simulink model "SRM_IOT"  (R2024b)
settings: Solver=VariableStepAuto  StartTime=0.0  StopTime=10.0  RelTol=1e-3
undefined symbols (not defined in the file): Ion, Lithium, sigbuilder_block
libraries: spsBreakerLib x120, spsSeriesRLCBranchLib x70, spsBatteryLib x42, spsIdealSwitchLib x33, spsVoltageMeasurementLib x27, slpidlib x17, spsMosfetLib x17, spsPWMGeneratorDCDCLib x11, spsDiodeLib x6, spsCurrentMeasurementLib x4, spsIGBTLib x2, spsThreePhaseSeriesRLCLoadLib x2
(part 1 of 5)
settings Model: SimulationMode=accelerator  Creator=Jatay  LastModifiedBy=Jatay

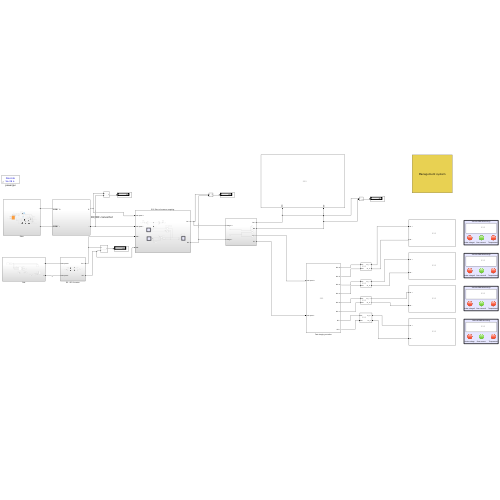
[thumbnail: Simulink's stored preview of the top-level diagram]
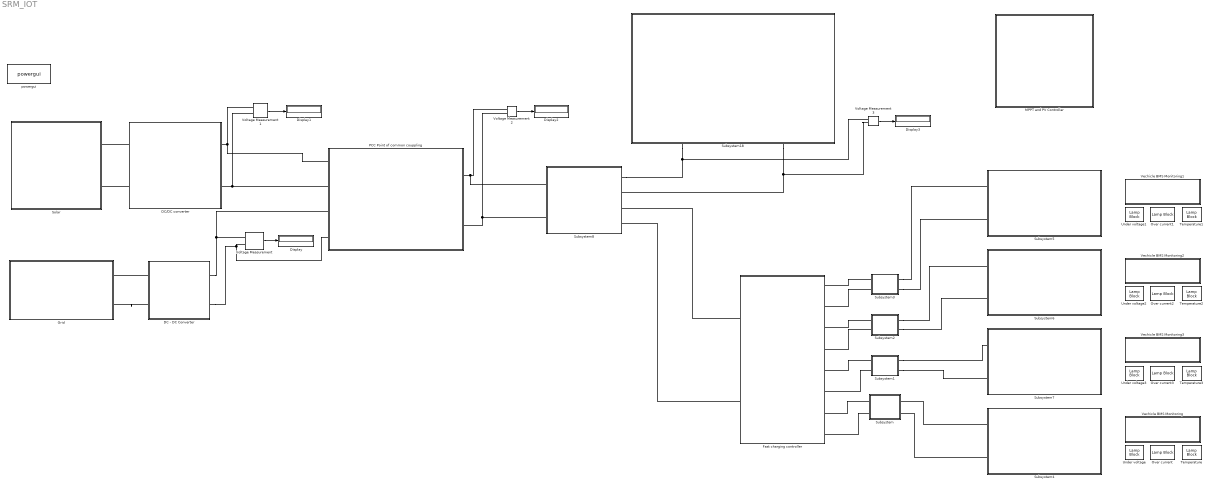
== system SRM_IOT ==
  DC - DC Converter : Subsystem
  DC/DC converter : Subsystem
  Display{,1..3} (4 alike) : Display
  Fast charging controller : Subsystem
      mask Display: image('FC.jpeg');
  Grid : Subsystem
  MPPT and PV Controller : Subsystem
      mask Display: disp('Management system')
  Over current{,1..3} (4 alike) : LampBlock  LabelPosition=Hide
  PCC Point of common couppling : Subsystem
  Solar : Subsystem
  Subsystem : Subsystem
      mask Display: image('plugin.jpeg');
  Subsystem1 : Subsystem
      mask Display: image('plugin.jpeg');
  Subsystem18 : Subsystem
      mask Display: image('swapping.webp');
  Subsystem2 : Subsystem
      mask Display: image('plugin.jpeg');
  Subsystem3 : Subsystem
      mask Display: image('plugin.jpeg');
  Subsystem4 : Subsystem
      mask Display: image('ev-1.jpeg');
  Subsystem5 : Subsystem
      mask Display: image('ev-1.jpeg');
  Subsystem6 : Subsystem
      mask Display: image('ev-1.jpeg');
  Subsystem7 : Subsystem
      mask Display: image('ev-1.jpeg');
  Subsystem8 : Subsystem
  Temperature{,1..3} (4 alike) : LampBlock  LabelPosition=Hide
  Under voltage{,1..3} (4 alike) : LampBlock  LabelPosition=Hide
  Vechicle BMS Monitoring : Subsystem
      mask Display: image('Dash_board.jpeg');
  Vechicle BMS Monitoring1 : Subsystem
      mask Display: image('Dash_board.jpeg');
  Vechicle BMS Monitoring2 : Subsystem
      mask Display: image('Dash_board.jpeg');
  Vechicle BMS Monitoring3 : Subsystem
      mask Display: image('Dash_board.jpeg');
  Voltage Measurement{,1..3} (4 alike) : spsVoltageMeasurementLib/Voltage Measurement  PhasorSimulation=off  OutputType=Complex  PSBequivalent=0
  powergui : sps_lib/powergui  Priority=1  SimulationMode=Discrete  SampleTime=5e-6  frequency=60  Iterations=50  frequencyindice=0  Pbase=100e6  ErrMax=1e-4  UnitsV=kV  UnitsW=MW  buscounter=0  FunctionMessages=off  echomessages=off  EnableUseOfTLC=off  CurrentSourceSwitches=off  DisableSnubberDevices=off  DisableRonSwitches=off  DisableVfSwitches=off  DisplayEquations=off  AutomaticDiscreteSolvers=off  SolverType=Tustin  Interpol=off  ExternalGateDelay=off  methode=off  Ts=0  x0status=blocks  SPID=off  SwTol=0  HookPort=off  NonlinearTolerance=1e-4  nMaxIteration=100  ContinueOnMaxIteration=off  RestoreLinks=warning  ResistiveCurrentMeasurement=off  Frange=[0:2:500]  Ylog=off  Xlog=on  ShowGrid=off  save=off  variable=ZData  structure=0  ZoomFFT=off  StartTime=0.0  cycles=1  DisplayStyle=1  fundamental=60  FreqAxis=off  MaxFrequency=1000  frequencyindicesteady=1  RmsSteady=1  display=off
  wires:
  Voltage Measurement/1 -> Display/1
  Voltage Measurement1/1 -> Display1/1
  Voltage Measurement2/1 -> Display2/1
  Voltage Measurement3/1 -> Display3/1
  connections:
  DC - DC Converter/LConn1 -- Grid/RConn1
  DC - DC Converter/RConn2 -- PCC Point of common couppling/LConn4 -- Voltage Measurement/LConn2
  DC - DC Converter/LConn2 -- Grid/RConn2
  DC - DC Converter/RConn1 -- PCC Point of common couppling/LConn3 -- Voltage Measurement/LConn1
  DC/DC converter/LConn2 -- Solar/RConn2
  DC/DC converter/LConn1 -- Solar/RConn1
  Voltage Measurement1/LConn1 -- PCC Point of common couppling/LConn1 -- DC/DC converter/RConn1
  Voltage Measurement1/LConn2 -- PCC Point of common couppling/LConn2 -- DC/DC converter/RConn2
  Voltage Measurement2/LConn1 -- Subsystem8/LConn1 -- PCC Point of common couppling/RConn1
  Voltage Measurement2/LConn2 -- PCC Point of common couppling/RConn2 -- Subsystem8/LConn2
  Subsystem18/LConn1 -- Subsystem8/RConn1 -- Voltage Measurement3/LConn1
  Subsystem18/LConn2 -- Subsystem8/RConn2 -- Voltage Measurement3/LConn2
  Subsystem3/RConn2 -- Subsystem5/LConn2
  Subsystem4/LConn1 -- Subsystem/RConn1
  Subsystem4/LConn2 -- Subsystem/RConn2
  Subsystem1/RConn1 -- Subsystem7/LConn1
  Subsystem2/RConn2 -- Subsystem6/LConn2
  Subsystem2/RConn1 -- Subsystem6/LConn1
  Subsystem3/RConn1 -- Subsystem5/LConn1
  Subsystem1/RConn2 -- Subsystem7/LConn2
  Fast charging controller/LConn2 -- Subsystem8/RConn3
  Fast charging controller/LConn1 -- Subsystem8/RConn4
  Subsystem3/LConn1 -- Fast charging controller/RConn8
  Subsystem3/LConn2 -- Fast charging controller/RConn7
  Subsystem2/LConn1 -- Fast charging controller/RConn6
  Subsystem2/LConn2 -- Fast charging controller/RConn5
  Subsystem1/LConn1 -- Fast charging controller/RConn4
  Subsystem1/LConn2 -- Fast charging controller/RConn3
  Subsystem/LConn1 -- Fast charging controller/RConn2
  Subsystem/LConn2 -- Fast charging controller/RConn1

== system SRM_IOT/DC - DC Converter ==
  C : spsSeriesRLCBranchLib/Series RLC Branch  LConnTagsString=__new0  RConnTagsString=__new0  BranchType=C  Resistance=0.01  Inductance=1e-3  SetiL0=off  InitialCurrent=0  Capacitance=1000e-6  Setx0=on  InitialVoltage=200  Measurements=None
  Diode : spsDiodeLib/Diode  Ron=0.001  Lon=0  Vf=1.1  IC=0  UseSnubber=off  Rs=500  Cs=250e-9  Measurements=off
  Diode2 : spsDiodeLib/Diode  Ron=0.001  Lon=0  Vf=0.7  IC=0  UseSnubber=off  Rs=500  Cs=250e-9  Measurements=off
  Display1 : Display
  Display2 : Display
  IGBT : spsIGBTLib/IGBT  Ron=0.001  Lon=0  Vf=1.1  Tf=1e-6  Tt=2e-6  IC=0  Rs=1e5  Cs=inf  Measurements=off
  Pulse Generator : DiscretePulseGenerator  PulseType=Time based  Period=10  PulseWidth=5
  RL : spsSeriesRLCBranchLib/Series RLC Branch  LConnTagsString=__new0  RConnTagsString=__new0  BranchType=RL  Resistance=0.05  Inductance=470e-6  SetiL0=off  InitialCurrent=0  Capacitance=1e-6  Setx0=off  InitialVoltage=0  Measurements=None
  Voltage Measurement1 : spsVoltageMeasurementLib/Voltage Measurement  PhasorSimulation=off  OutputType=Complex  PSBequivalent=0
  Voltage Measurement2 : spsVoltageMeasurementLib/Voltage Measurement  PhasorSimulation=off  OutputType=Complex  PSBequivalent=0
  DC + : PMIOPort  Side=Right
  solar panel + : PMIOPort  Port=2  Side=Left
  solar panel - : PMIOPort  Port=3  Side=Left
  DC - : PMIOPort  Port=4  Side=Right
  wires:
  Pulse Generator/1 -> IGBT/1
  Voltage Measurement1/1 -> Display1/1
  Voltage Measurement2/1 -> Display2/1
  connections:
  DC +/RConn1 -- Diode/RConn1 -- Voltage Measurement2/LConn1
  Diode2/RConn1 -- C/LConn1 -- RL/LConn1
  Diode/LConn1 -- RL/RConn1 -- IGBT/LConn1
  Diode2/LConn1 -- solar panel +/RConn1 -- Voltage Measurement1/LConn1
  DC -/RConn1 -- C/RConn1 -- Voltage Measurement1/LConn2 -- solar panel -/RConn1 -- IGBT/RConn1 -- Voltage Measurement2/LConn2

== system SRM_IOT/DC//DC converter ==
  DC - DC Converter : Subsystem
  DC bus : Subsystem
  Display : Display
  Voltage Measurement : spsVoltageMeasurementLib/Voltage Measurement  PhasorSimulation=off  OutputType=Complex  PSBequivalent=0
  Voltage Measurement2 : spsVoltageMeasurementLib/Voltage Measurement  PhasorSimulation=off  OutputType=Complex  PSBequivalent=0
  solar + : PMIOPort  Side=Left
  solar - : PMIOPort  Port=2  Side=Left
  + : PMIOPort  Port=3  Side=Right
  - : PMIOPort  Port=4  Side=Right
  tag scope: solar_controller=global
  wires:
  Voltage Measurement2/1 -> [solar_controller]
  Voltage Measurement/1 -> Display/1
  connections:
  DC - DC Converter/RConn1 -- DC bus/LConn1
  solar +/RConn1 -- DC - DC Converter/LConn1 -- Voltage Measurement2/LConn1
  DC - DC Converter/LConn2 -- Voltage Measurement2/LConn2 -- solar -/RConn1
  DC - DC Converter/RConn2 -- DC bus/LConn2
  -/RConn1 -- DC bus/RConn2 -- Voltage Measurement/LConn2
  Voltage Measurement/LConn1 -- DC bus/RConn1 -- +/RConn1

== system SRM_IOT/Fast charging controller ==
  note: Solar
  Fast charging Switching controller : Subsystem
  Ideal Switch{,1..3} (4 alike) : spsIdealSwitchLib/Ideal Switch  Ron=0.001  Lon=0  IC=0  Rs=1e5  Cs=inf  Measurements=off
  solar panel - : PMIOPort  Side=Left
  solar panel + : PMIOPort  Port=2  Side=Left
  DC + : PMIOPort  Port=3  Side=Right
  DC - : PMIOPort  Port=4  Side=Right
  DC +1 : PMIOPort  Port=5  Side=Right
  DC +2 : PMIOPort  Port=6  Side=Right
  DC +3 : PMIOPort  Port=7  Side=Right
  DC +4 : PMIOPort  Port=8  Side=Right
  DC +5 : PMIOPort  Port=9  Side=Right
  DC +6 : PMIOPort  Port=10  Side=Right
  wires:
  [gg1] -> Ideal Switch3/1
  [gg2] -> Ideal Switch2/1
  [gg3] -> Ideal Switch1/1
  [gg4] -> Ideal Switch/1
  connections:
  Ideal Switch3/LConn1 -- Ideal Switch2/LConn1 -- Ideal Switch1/LConn1 -- Ideal Switch/LConn1 -- solar panel +/RConn1
  solar panel -/RConn1 -- DC +5/RConn1 -- DC +4/RConn1 -- DC +2/RConn1 -- DC -/RConn1
  Ideal Switch3/RConn1 -- DC +/RConn1
  Ideal Switch2/RConn1 -- DC +1/RConn1
  Ideal Switch1/RConn1 -- DC +3/RConn1
  Ideal Switch/RConn1 -- DC +6/RConn1

== system SRM_IOT/Grid ==
  Display : Display
  Grid : spsThreePhaseSourceLib/Three-Phase Source  InternalConnection=Yg  VoltagePhases=off  Voltage=380  PhaseAngle=0  Voltage_phases=[25e3 25e3 25e3]/sqrt(3)  PhaseAngles_phases=[0 -120 +120]  Frequency=50  NonIdealSource=on  SpecifyImpedance=on  Resistance=0.8929  Inductance=16.58e-3  ShortCircuitLevel=100e6  BaseVoltage=380  XRratio=7  BusType=swing  Pref=10e3  Qref=0  Prefabc=[10e3, 10e3, 10e3]  Qrefabc=[0, 0, 0]  Qmin=-inf  Qmax=inf
  LOAD1 : spsThreePhaseSeriesRLCLoadLib/Three-Phase Series RLC Load  LConnTagsString=A|B|C  Configuration=Y (grounded)  NominalVoltage=380  Vabc=[1e3 1e3 1e3]  Vabcp=[1e3 1e3 1e3]  NominalFrequency=50  UnbalancedPower=off  ActivePower=1e3  InductivePower=0  CapacitivePower=0  Pabc=[10e3 9e3 11e3]  QLabc=[100 90 110]  QCabc=[100 90 110]  Pabcp=[10e3 9e3 11e3]  QLabcp=[100 90 110]  QCabcp=[100 90 110]  Measurements=None  LoadType=constant Z
  Measurement : spsThreePhaseVIMeasurementLib/Three-Phase V-I Measurement  VoltageMeasurement=phase-to-phase  SetLabelV=on  LabelV=Vabc_grid  Vpu=off  VpuLL=off  CurrentMeasurement=yes  SetLabelI=on  LabelI=Iabc_grid  Ipu=off  Pbase=100e6  Vbase=500e3  OutputType=Complex  PhasorSimulation=off  PSBequivalent=0
  Mux : Mux  Inputs=2
  Repeating Sequence Stair : simulink/Sources/Repeating Sequence Stair  OutValues=[0 0 1 1 0].'  tsamp=0.1  OutMin=[]  OutMax=[]  OutDataTypeStr=double  OutputDataTypeScalingMode=double  OutDataType=fixdt(0,8)  ConRadixGroup=Best Precision: Vector-wise  OutScaling=2^-12
  Scope : Scope
  Scope1 : Scope
  Scope2 : Scope  NumInputPorts=2
  V2G & G2V results : Scope  NumInputPorts=3
  Voltage Measurement : spsVoltageMeasurementLib/Voltage Measurement  PhasorSimulation=off  OutputType=Complex  PSBequivalent=0
  Wall charger Connection Box : Subsystem
  + : PMIOPort  Side=Right
  +1 : PMIOPort  Port=2  Side=Right
  tag scope: Control=global
  wires:
  [Control] -> Wall charger Connection Box/1(Control)
  Mux/1 -> V2G & G2V results/3
  [Vabc_grid] -> V2G & G2V results/1
  [Vabc_inv] -> V2G & G2V results/2
  Repeating Sequence Stair/1 -> [Control], Scope1/1
  [Vabc_inv] -> Mux/2
  [Iabc_out] -> Scope2/2
  [Iabc_inv] -> Scope/1
  [Vabc_out] -> Scope2/1
  Voltage Measurement/1 -> Display/1
  [Vabc_grid] -> Mux/1
  connections:
  Wall charger Connection Box/RConn2 -- Voltage Measurement/LConn2 -- +1/RConn1
  Grid/RConn1 -- Measurement/LConn1
  Grid/RConn3 -- Measurement/LConn3
  Wall charger Connection Box/RConn1 -- Voltage Measurement/LConn1 -- +/RConn1
  Grid/RConn2 -- Measurement/LConn2
  LOAD1/LConn3 -- Measurement/RConn3 -- Wall charger Connection Box/LConn3
  Measurement/RConn2 -- LOAD1/LConn2 -- Wall charger Connection Box/LConn2
  Measurement/RConn1 -- LOAD1/LConn1 -- Wall charger Connection Box/LConn1

== system SRM_IOT/MPPT and PV Controller ==
  Inverter controller : Subsystem
  Swapping battery controller : Subsystem

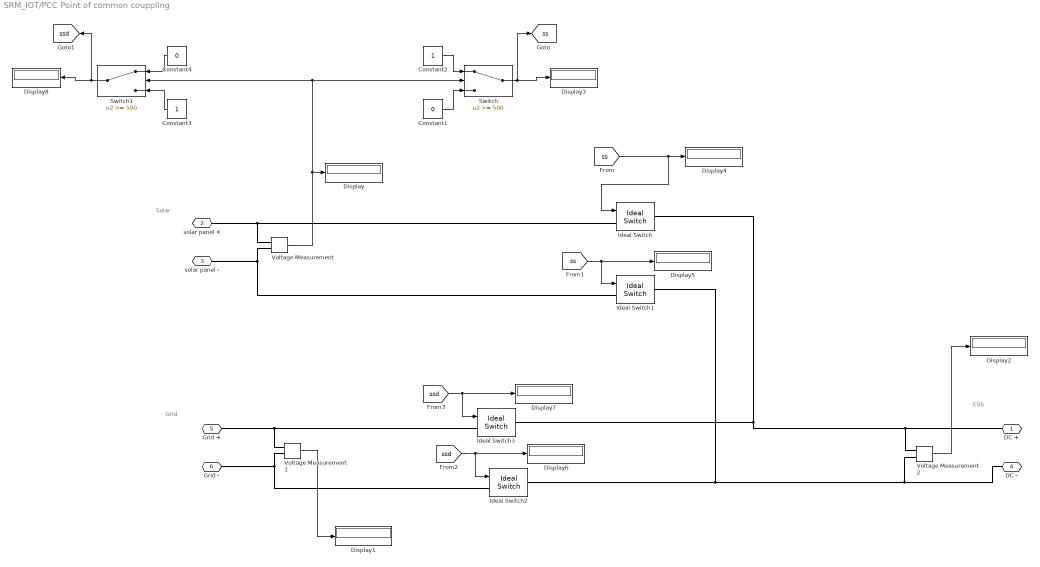
== system SRM_IOT/PCC Point of common couppling ==
  note: ESS
  note: Grid
  note: Solar
  Constant1 : Constant  Value=0
  Constant2 : Constant
  Constant3 : Constant
  Constant4 : Constant  Value=0
  Display{,1..8} (9 alike) : Display
  Ideal Switch{,1..3} (4 alike) : spsIdealSwitchLib/Ideal Switch  Ron=0.001  Lon=0  IC=0  Rs=1e5  Cs=inf  Measurements=off
  Switch : Switch  Threshold=500  SaturateOnIntegerOverflow=off  InputSameDT=off
  Switch1 : Switch  Threshold=500  SaturateOnIntegerOverflow=off  InputSameDT=off
  Voltage Measurement : spsVoltageMeasurementLib/Voltage Measurement  PhasorSimulation=off  OutputType=Complex  PSBequivalent=0
  Voltage Measurement1 : spsVoltageMeasurementLib/Voltage Measurement  PhasorSimulation=off  OutputType=Complex  PSBequivalent=0
  Voltage Measurement2 : spsVoltageMeasurementLib/Voltage Measurement  PhasorSimulation=off  OutputType=Complex  PSBequivalent=0
  DC + : PMIOPort  Side=Right
  solar panel + : PMIOPort  Port=2  Side=Left
  solar panel - : PMIOPort  Port=3  Side=Left
  DC - : PMIOPort  Port=4  Side=Right
  Grid + : PMIOPort  Port=5  Side=Left
  Grid - : PMIOPort  Port=6  Side=Left
  tag scope: ss=global, ssd=global
  wires:
  Voltage Measurement1/1 -> Display1/1
  Voltage Measurement2/1 -> Display2/1
  Switch/1 -> Display3/1, [ss]
  Constant2/1 -> Switch/1
  Constant1/1 -> Switch/3
  [ss] -> Ideal Switch/1, Display4/1
  [ss] -> Ideal Switch1/1, Display5/1
  [ssd] -> Ideal Switch2/1, Display6/1
  [ssd] -> Ideal Switch3/1, Display7/1
  Constant3/1 -> Switch1/3
  Voltage Measurement/1 -> Switch/2, Switch1/2, Display/1
  Constant4/1 -> Switch1/1
  Switch1/1 -> Display8/1, [ssd]
  connections:
  Voltage Measurement2/LConn2 -- Ideal Switch1/RConn1 -- Ideal Switch2/RConn1 -- DC -/RConn1
  Voltage Measurement2/LConn1 -- Ideal Switch3/RConn1 -- Ideal Switch/RConn1 -- DC +/RConn1
  Voltage Measurement/LConn1 -- solar panel +/RConn1 -- Ideal Switch/LConn1
  Voltage Measurement/LConn2 -- Ideal Switch1/LConn1 -- solar panel -/RConn1
  Voltage Measurement1/LConn2 -- Ideal Switch2/LConn1 -- Grid -/RConn1
  Grid +/RConn1 -- Ideal Switch3/LConn1 -- Voltage Measurement1/LConn1

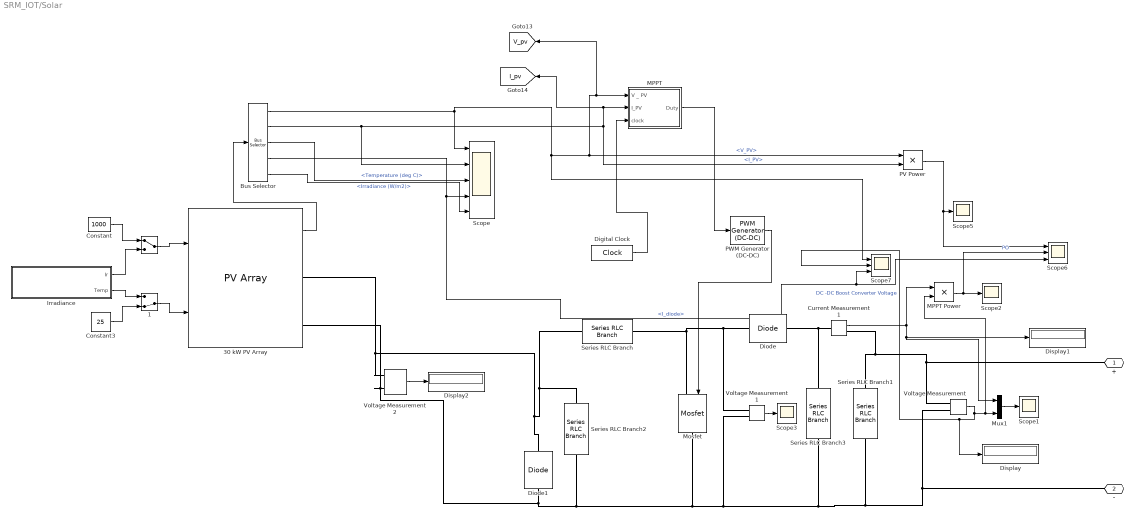
== system SRM_IOT/Solar ==
  "      " : ManualSwitch
  "      1" : ManualSwitch  CurrentSetting=0
  30 kW PV Array : spsPVArrayLib/PV Array  Npar=15  Nser=10  PlotType=array @ 1000 W/m2 & specified temperatures  S_vec="[ 1000  500  100 ]"  Temp_C_vec="[ 45 25  ]"  ModuleName=User-defined  PlotWhenSelected=off  Pm=213.15  Ncell=60  Voc=48  Isc=7.84  Vm=29  Im=7.35  beta_Voc_pc=-0.36099  alpha_Isc_pc=0.102  beta_Voc=-0.17328  alpha_Isc=0.0079968  IL=8.2285  I0=2.9956e-10  nI=1.2955  Rsh=7353.5939  Rs=2.0228  RobustModel=off  RobustCellTemperature=25  BAL=on  Tc=1e-6  Tfilter=5e-5
  Bus Selector : BusSelector  OutputSignals=V_PV,I_PV,Temperature (deg C),I_diode,Irradiance (W/m2)
  Constant : Constant  Value=1000
  Constant3 : Constant  Value=25
  Current Measurement1 : spsCurrentMeasurementLib/Current Measurement  PhasorSimulation=off  OutputType=Complex  PSBequivalent=0
  Digital Clock : DigitalClock  SampleTime=0.001
  Diode : spsDiodeLib/Diode  Ron=0.5  Lon=0  Vf=0.7  IC=0  UseSnubber=0  Rs=1e5  Cs=250e-9  Measurements=off
  Diode1 : spsDiodeLib/Diode  Ron=0.5  Lon=0  Vf=0.7  IC=0  UseSnubber=0  Rs=1e5  Cs=250e-9  Measurements=off
  Display : Display
  Display1 : Display
  Display2 : Display
  "Irradiance " : Subsystem  Tag=STV Subsys  LoadFcn=sigbuilder_block('load');  StartFcn=sigbuilder_block('start');  StopFcn=sigbuilder_block('stop');  ClipboardFcn=sigbuilder_block('clipboard');  mask(Sigbuilder block){tuvar=[0:10]}
      mask help: Sigbuilder GUI
      mask init:
      | if ~strcmp(get_param(bdroot(gcbh),'SimulationStatus'),'stopped') tuvar = sigbuilder_block('maskInit'); end
      settings: CopyFcn=sigbuilder_block('copy');  DeleteFcn=sigbuilder_block('delete');  ModelCloseFcn=sigbuilder_block('modelClose');  PreSaveFcn=sigbuilder_block('preSave');  PauseFcn=sigbuilder_block('pause')  ContinueFcn=sigbuilder_block('continue')  NameChangeFcn=sigbuilder_block('namechange');  OpenFcn=sigbuilder_block('open',[5.4 30 1141.2 507.6 ]);  CloseFcn=sigbuilder_block('close');
      mask Display: plot(0, 0, 100, 100,[2, 2, 32, 32, 2], [68, 8, 8, 68, 68],[32, 2], [38, 38], [32, 19, 2],[53, 60, 44], [32, 17, 17, 2],[16, 16, 31, 31]);txt = getActiveGroup(gcbh);text(2, 100, txt,'verticalAlignment', 'top');
  MPPT : Subsystem
  MPPT Power : Product
  Mosfet : spsMosfetLib/Mosfet  Ron=0.1  Lon=0  Rd=0.01  Vfd=0.7  IC=0  Rs=1e5  Cs=inf  Measurements=off
  Mux1 : Mux  Inputs=2
  PV Power : Product
  PWM Generator (DC-DC) : spsPWMGeneratorDCDCLib/PWM Generator (DC-DC)  Fsw=1500  Ts=0
  Scope : Scope  NumInputPorts=5
  Scope{1..3,5} (4 alike) : Scope
  Scope6 : Scope  NumInputPorts=3
  Scope7 : Scope  NumInputPorts=3
  Series RLC Branch : spsSeriesRLCBranchLib/Series RLC Branch  LConnTagsString=__new0  RConnTagsString=__new0  BranchType=L  Resistance=0.001  Inductance=0.4e-1  SetiL0=off  InitialCurrent=0  Capacitance=1e-6  Setx0=off  InitialVoltage=0  Measurements=None
  Series RLC Branch1 : spsSeriesRLCBranchLib/Series RLC Branch  LConnTagsString=__new0  RConnTagsString=__new0  BranchType=R  Resistance=11  Inductance=0.1  SetiL0=off  InitialCurrent=0  Capacitance=100e-6  Setx0=off  InitialVoltage=0  Measurements=None
  Series RLC Branch2 : spsSeriesRLCBranchLib/Series RLC Branch  LConnTagsString=__new0  RConnTagsString=__new0  BranchType=C  Resistance=6  Inductance=0.1  SetiL0=off  InitialCurrent=0  Capacitance=700e-5  Setx0=off  InitialVoltage=0  Measurements=None
  Series RLC Branch3 : spsSeriesRLCBranchLib/Series RLC Branch  LConnTagsString=__new0  RConnTagsString=__new0  BranchType=C  Resistance=6  Inductance=0.1  SetiL0=off  InitialCurrent=0  Capacitance=1000e-5  Setx0=off  InitialVoltage=0  Measurements=None
  Voltage Measurement : spsVoltageMeasurementLib/Voltage Measurement  PhasorSimulation=off  OutputType=Complex  PSBequivalent=0
  Voltage Measurement1 : spsVoltageMeasurementLib/Voltage Measurement  PhasorSimulation=off  OutputType=Complex  PSBequivalent=0
  Voltage Measurement2 : spsVoltageMeasurementLib/Voltage Measurement  PhasorSimulation=off  OutputType=Complex  PSBequivalent=0
  + : PMIOPort  Side=Right
  - : PMIOPort  Port=2  Side=Right
  tag scope: I_pv=global, V_pv=global
  wires:
  Voltage Measurement/1 -> MPPT Power/2, Mux1/2, Display/1, Scope7/2  "DC -DC Boost Converter Voltage"
  PWM Generator (DC-DC)/1 -> Mosfet/1
  Mux1/1 -> Scope1/1
  MPPT Power/1 -> Scope6/2, Scope2/1  "PO"
  Current Measurement1/1 -> MPPT Power/1, Display1/1, Mux1/1
  Voltage Measurement1/1 -> Scope3/1
  Bus Selector/3 -> Scope/3  "<Temperature (deg C)>"
  Bus Selector/4 -> Scope6/3, Scope7/3, Scope/4  "<I_diode>"
  Digital Clock/1 -> MPPT/3(clock)
  MPPT/1(Duty) -> PWM Generator (DC-DC)/1
  PV Power/1 -> Scope6/1, Scope5/1
  "Irradiance "/2(Temp) -> "      1"/1
  Constant3/1 -> "      1"/2
  "Irradiance "/1(Ir) -> "      "/2
  Constant/1 -> "      "/1
  "      "/1 -> 30 kW PV Array/1
  "      1"/1 -> 30 kW PV Array/2
  Voltage Measurement2/1 -> Display2/1
  30 kW PV Array/1 -> Bus Selector/1
  Bus Selector/2 -> Scope/2, MPPT/2(I_PV), [I_pv], PV Power/2  "<I_PV>"
  Bus Selector/5 -> Scope/5  "<Irradiance (W/m2)>"
  Bus Selector/1 -> Scope7/1, PV Power/1, [V_pv], MPPT/1("V _ PV "), Scope/1  "<V_PV>"
  connections:
  Voltage Measurement/LConn2 -- Voltage Measurement2/LConn2 -- 30 kW PV Array/RConn2 -- Diode1/LConn1 -- Series RLC Branch2/RConn1 -- Mosfet/RConn1 -- Voltage Measurement1/LConn2 -- Series RLC Branch3/RConn1 -- Series RLC Branch1/RConn1 -- -/RConn1
  Current Measurement1/RConn1 -- Series RLC Branch1/LConn1 -- Voltage Measurement/LConn1 -- +/RConn1
  Diode/RConn1 -- Series RLC Branch3/LConn1 -- Current Measurement1/LConn1
  Voltage Measurement1/LConn1 -- Series RLC Branch/RConn1 -- Mosfet/LConn1 -- Diode/LConn1
  Series RLC Branch2/LConn1 -- Voltage Measurement2/LConn1 -- 30 kW PV Array/RConn1 -- Diode1/RConn1 -- Series RLC Branch/LConn1

== system SRM_IOT/Subsystem ==
  1 : spsMosfetLib/Mosfet  Ron=0.1  Lon=0  Rd=0.01  Vfd=0  IC=0  Rs=1e5  Cs=inf  Measurements=off
  2 : spsMosfetLib/Mosfet  Ron=0.1  Lon=0  Rd=0.01  Vfd=0  IC=0  Rs=1e5  Cs=inf  Measurements=off
  Constant : Constant
  Control : Subsystem
  Ideal Switch : spsIdealSwitchLib/Ideal Switch  Ron=0.001  Lon=0  IC=0  Rs=1e5  Cs=inf  Measurements=off
  Series RLC Branch : spsSeriesRLCBranchLib/Series RLC Branch  LConnTagsString=__new0  RConnTagsString=__new0  BranchType=RL  Resistance=0.05  Inductance=5.76e-3  SetiL0=off  InitialCurrent=0  Capacitance=1e-6  Setx0=off  InitialVoltage=0  Measurements=None
  Series RLC Branch1 : spsSeriesRLCBranchLib/Series RLC Branch  LConnTagsString=__new0  RConnTagsString=__new0  BranchType=R  Resistance=5  Inductance=5.76e-4  SetiL0=off  InitialCurrent=0  Capacitance=1e-6  Setx0=off  InitialVoltage=0  Measurements=None
  Series RLC Branch2 : spsSeriesRLCBranchLib/Series RLC Branch  LConnTagsString=__new0  RConnTagsString=__new0  BranchType=RC  Resistance=0.001  Inductance=5.76e-4  SetiL0=off  InitialCurrent=0  Capacitance=1000e-6  Setx0=off  InitialVoltage=0  Measurements=None
  bb - : PMIOPort  Side=Left
  bb + : PMIOPort  Port=2  Side=Left
  vv_1 + : PMIOPort  Port=3  Side=Right
  vv_2 - : PMIOPort  Port=4  Side=Right
  wires:
  [Mosfet_1] -> 1/1
  [Mosfet_2] -> 2/1
  Constant/1 -> Ideal Switch/1
  connections:
  Series RLC Branch2/LConn1 -- Series RLC Branch1/LConn1 -- Ideal Switch/RConn1 -- 1/LConn1
  2/RConn1 -- vv_2 -/RConn1 -- bb -/RConn1 -- Series RLC Branch1/RConn1 -- Series RLC Branch2/RConn1
  1/RConn1 -- 2/LConn1 -- Series RLC Branch/LConn1
  Series RLC Branch/RConn1 -- vv_1 +/RConn1
  bb +/RConn1 -- Ideal Switch/LConn1

== system SRM_IOT/Subsystem1 ==
  1 : spsMosfetLib/Mosfet  Ron=0.1  Lon=0  Rd=0.01  Vfd=0  IC=0  Rs=1e5  Cs=inf  Measurements=off
  2 : spsMosfetLib/Mosfet  Ron=0.1  Lon=0  Rd=0.01  Vfd=0  IC=0  Rs=1e5  Cs=inf  Measurements=off
  Constant : Constant
  Control : Subsystem
  Ideal Switch : spsIdealSwitchLib/Ideal Switch  Ron=0.001  Lon=0  IC=0  Rs=1e5  Cs=inf  Measurements=off
  Series RLC Branch : spsSeriesRLCBranchLib/Series RLC Branch  LConnTagsString=__new0  RConnTagsString=__new0  BranchType=RL  Resistance=0.05  Inductance=5.76e-3  SetiL0=off  InitialCurrent=0  Capacitance=1e-6  Setx0=off  InitialVoltage=0  Measurements=None
  Series RLC Branch1 : spsSeriesRLCBranchLib/Series RLC Branch  LConnTagsString=__new0  RConnTagsString=__new0  BranchType=R  Resistance=5  Inductance=5.76e-4  SetiL0=off  InitialCurrent=0  Capacitance=1e-6  Setx0=off  InitialVoltage=0  Measurements=None
  Series RLC Branch2 : spsSeriesRLCBranchLib/Series RLC Branch  LConnTagsString=__new0  RConnTagsString=__new0  BranchType=RC  Resistance=0.001  Inductance=5.76e-4  SetiL0=off  InitialCurrent=0  Capacitance=1000e-6  Setx0=off  InitialVoltage=0  Measurements=None
  bb - : PMIOPort  Side=Left
  bb + : PMIOPort  Port=2  Side=Left
  vv_1 + : PMIOPort  Port=3  Side=Right
  vv_2 - : PMIOPort  Port=4  Side=Right
  wires:
  [Mosfet_22] -> 1/1
  [Mosfet_222] -> 2/1
  Constant/1 -> Ideal Switch/1
  connections:
  Series RLC Branch2/LConn1 -- Series RLC Branch1/LConn1 -- Ideal Switch/RConn1 -- 1/LConn1
  bb -/RConn1 -- Series RLC Branch1/RConn1 -- Series RLC Branch2/RConn1 -- 2/RConn1 -- vv_2 -/RConn1
  1/RConn1 -- Series RLC Branch/LConn1 -- 2/LConn1
  Series RLC Branch/RConn1 -- vv_1 +/RConn1
  bb +/RConn1 -- Ideal Switch/LConn1

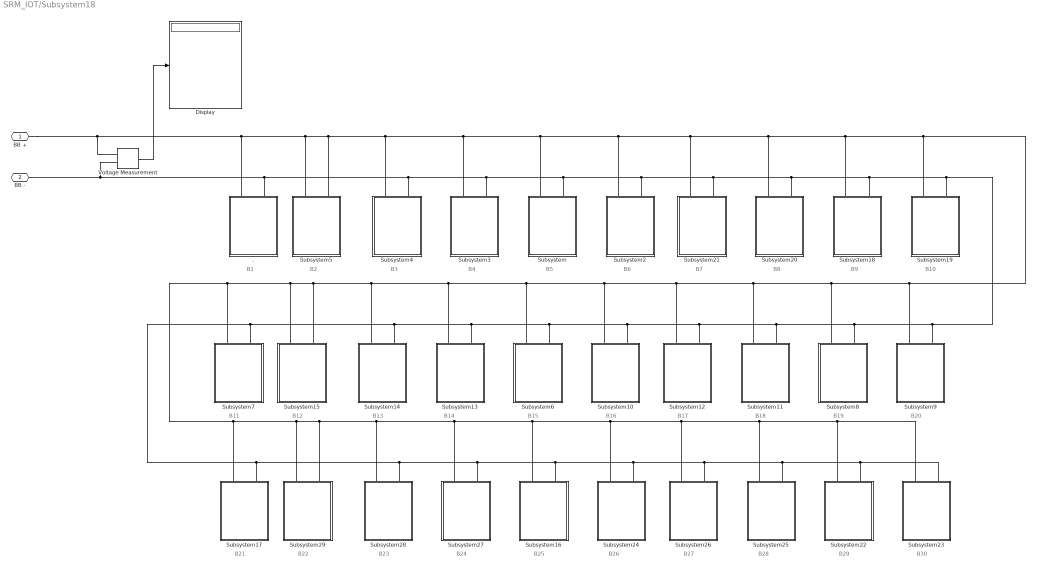
== system SRM_IOT/Subsystem18 ==
  note: B1
  note: B2
  note: B3
  note: B4
  note: B5
  note: B6
  note: B13
  note: B14
  note: B15
  note: B16
  note: B17
  note: B18
  note: B19
  note: B20
  note: B21
  note: B22
  note: B7
  note: B8
  note: B9
  note: B10
  note: B11
  note: B12
  note: B23
  note: B24
  note: B25
  note: B26
  note: B27
  note: B28
  note: B29
  note: B30
  . : Subsystem
  Display : Display
      settings: Decimation=2
  Subsystem : Subsystem
  Subsystem10 : Subsystem
  Subsystem11 : Subsystem
  Subsystem12 : Subsystem
  Subsystem13 : Subsystem
  Subsystem14 : Subsystem
  Subsystem15 : Subsystem
  Subsystem16 : Subsystem
  Subsystem17 : Subsystem
  Subsystem18 : Subsystem
  Subsystem19 : Subsystem
  Subsystem2 : Subsystem
  Subsystem20 : Subsystem
  Subsystem21 : Subsystem
  Subsystem22 : Subsystem
  Subsystem23 : Subsystem
  Subsystem24 : Subsystem
  Subsystem25 : Subsystem
  Subsystem26 : Subsystem
  Subsystem27 : Subsystem
  Subsystem28 : Subsystem
  Subsystem29 : Subsystem
  Subsystem3 : Subsystem
  Subsystem4 : Subsystem
  Subsystem5 : Subsystem
  Subsystem6 : Subsystem
  Subsystem7 : Subsystem
  Subsystem8 : Subsystem
  Subsystem9 : Subsystem
  Voltage Measurement : spsVoltageMeasurementLib/Voltage Measurement  PhasorSimulation=off  OutputType=Complex  PSBequivalent=0
  BB + : PMIOPort  Side=Left
  BB - : PMIOPort  Port=2  Side=Left
  wires:
  Voltage Measurement/1 -> Display/1
  connections:
  ./RConn2 -- Subsystem21/RConn2 -- Subsystem19/RConn2 -- Subsystem9/RConn2 -- Subsystem8/RConn2 -- Subsystem11/RConn2 -- Subsystem12/RConn2 -- Subsystem10/RConn2 -- Subsystem6/RConn2 -- Subsystem13/RConn2 -- Subsystem14/RConn2 -- Subsystem7/RConn2 -- Subsystem17/RConn2 -- Subsystem28/RConn2 -- Subsystem27/RConn2 -- Subsystem16/RConn2 -- Subsystem26/RConn2 -- Subsystem23/RConn2 -- Subsystem22/RConn2 -- Subsystem25/RConn2 -- Subsystem24/RConn2 -- Subsystem18/RConn2 -- Subsystem20/RConn2 -- Subsystem2/RConn2 -- Subsystem/RConn2 -- Subsystem3/RConn2 -- Subsystem4/RConn2 -- Voltage Measurement/LConn2 -- BB -/RConn1
  Subsystem10/RConn1 -- Subsystem7/RConn1 -- Subsystem17/RConn1 -- Subsystem29/RConn1 -- Subsystem29/RConn2 -- Subsystem28/RConn1 -- Subsystem27/RConn1 -- Subsystem16/RConn1 -- Subsystem26/RConn1 -- Subsystem25/RConn1 -- Subsystem22/RConn1 -- Subsystem23/RConn1 -- Subsystem24/RConn1 -- Subsystem15/RConn1 -- Subsystem15/RConn2 -- Subsystem14/RConn1 -- Subsystem13/RConn1 -- Subsystem6/RConn1 -- Subsystem12/RConn1 -- Subsystem11/RConn1 -- Subsystem8/RConn1 -- Subsystem20/RConn1 -- Voltage Measurement/LConn1 -- BB +/RConn1 -- ./RConn1 -- Subsystem5/RConn1 -- Subsystem5/RConn2 -- Subsystem4/RConn1 -- Subsystem3/RConn1 -- Subsystem/RConn1 -- Subsystem2/RConn1 -- Subsystem21/RConn1 -- Subsystem18/RConn1 -- Subsystem19/RConn1 -- Subsystem9/RConn1

== system SRM_IOT/Subsystem2 ==
  1 : spsMosfetLib/Mosfet  Ron=0.1  Lon=0  Rd=0.01  Vfd=0  IC=0  Rs=1e5  Cs=inf  Measurements=off
  2 : spsMosfetLib/Mosfet  Ron=0.1  Lon=0  Rd=0.01  Vfd=0  IC=0  Rs=1e5  Cs=inf  Measurements=off
  Constant : Constant
  Control : Subsystem
  Ideal Switch : spsIdealSwitchLib/Ideal Switch  Ron=0.001  Lon=0  IC=0  Rs=1e5  Cs=inf  Measurements=off
  Series RLC Branch : spsSeriesRLCBranchLib/Series RLC Branch  LConnTagsString=__new0  RConnTagsString=__new0  BranchType=RL  Resistance=0.05  Inductance=5.76e-3  SetiL0=off  InitialCurrent=0  Capacitance=1e-6  Setx0=off  InitialVoltage=0  Measurements=None
  Series RLC Branch1 : spsSeriesRLCBranchLib/Series RLC Branch  LConnTagsString=__new0  RConnTagsString=__new0  BranchType=R  Resistance=5  Inductance=5.76e-4  SetiL0=off  InitialCurrent=0  Capacitance=1e-6  Setx0=off  InitialVoltage=0  Measurements=None
  Series RLC Branch2 : spsSeriesRLCBranchLib/Series RLC Branch  LConnTagsString=__new0  RConnTagsString=__new0  BranchType=RC  Resistance=0.001  Inductance=5.76e-4  SetiL0=off  InitialCurrent=0  Capacitance=1000e-6  Setx0=off  InitialVoltage=0  Measurements=None
  bb - : PMIOPort  Side=Left
  bb + : PMIOPort  Port=2  Side=Left
  vv_1 + : PMIOPort  Port=3  Side=Right
  vv_2 - : PMIOPort  Port=4  Side=Right
  wires:
  [Mosfet_33] -> 1/1
  [Mosfet_333] -> 2/1
  Constant/1 -> Ideal Switch/1
  connections:
  Series RLC Branch2/LConn1 -- Series RLC Branch1/LConn1 -- Ideal Switch/RConn1 -- 1/LConn1
  bb -/RConn1 -- Series RLC Branch1/RConn1 -- Series RLC Branch2/RConn1 -- 2/RConn1 -- vv_2 -/RConn1
  1/RConn1 -- Series RLC Branch/LConn1 -- 2/LConn1
  Series RLC Branch/RConn1 -- vv_1 +/RConn1
  bb +/RConn1 -- Ideal Switch/LConn1

== system SRM_IOT/Subsystem3 ==
  1 : spsMosfetLib/Mosfet  Ron=0.1  Lon=0  Rd=0.01  Vfd=0  IC=0  Rs=1e5  Cs=inf  Measurements=off
  2 : spsMosfetLib/Mosfet  Ron=0.1  Lon=0  Rd=0.01  Vfd=0  IC=0  Rs=1e5  Cs=inf  Measurements=off
  Control : Subsystem
  Display : Display
  Series RLC Branch : spsSeriesRLCBranchLib/Series RLC Branch  LConnTagsString=__new0  RConnTagsString=__new0  BranchType=RL  Resistance=0.05  Inductance=5.76e-3  SetiL0=off  InitialCurrent=0  Capacitance=1e-6  Setx0=off  InitialVoltage=0  Measurements=None
  Series RLC Branch1 : spsSeriesRLCBranchLib/Series RLC Branch  LConnTagsString=__new0  RConnTagsString=__new0  BranchType=R  Resistance=5  Inductance=5.76e-4  SetiL0=off  InitialCurrent=0  Capacitance=1e-6  Setx0=off  InitialVoltage=0  Measurements=None
  Series RLC Branch2 : spsSeriesRLCBranchLib/Series RLC Branch  LConnTagsString=__new0  RConnTagsString=__new0  BranchType=RC  Resistance=0.001  Inductance=5.76e-4  SetiL0=off  InitialCurrent=0  Capacitance=1000e-6  Setx0=off  InitialVoltage=0  Measurements=None
  Voltage Measurement : spsVoltageMeasurementLib/Voltage Measurement  PhasorSimulation=off  OutputType=Complex  PSBequivalent=0
  bb - : PMIOPort  Side=Left
  bb + : PMIOPort  Port=2  Side=Left
  vv_1 + : PMIOPort  Port=3  Side=Right
  vv_2 - : PMIOPort  Port=4  Side=Right
  wires:
  [Mosfet_44] -> 1/1
  [Mosfet_444] -> 2/1
  Voltage Measurement/1 -> Display/1
  connections:
  Series RLC Branch2/LConn1 -- Series RLC Branch1/LConn1 -- bb +/RConn1 -- 1/LConn1
  bb -/RConn1 -- Series RLC Branch1/RConn1 -- Series RLC Branch2/RConn1 -- 2/RConn1 -- Voltage Measurement/LConn2 -- vv_2 -/RConn1
  1/RConn1 -- Series RLC Branch/LConn1 -- 2/LConn1
  Series RLC Branch/RConn1 -- Voltage Measurement/LConn1 -- vv_1 +/RConn1

== system SRM_IOT/Subsystem4 ==
  Constant : Constant  Value=300
  Current Measurement : spsCurrentMeasurementLib/Current Measurement  PhasorSimulation=off  OutputType=Complex  PSBequivalent=0
  Display : Display
  Display1 : Display
  Series RLC Branch : spsSeriesRLCBranchLib/Series RLC Branch  LConnTagsString=__new0  RConnTagsString=__new0  BranchType=R  Resistance=5  Inductance=1e-3  SetiL0=off  InitialCurrent=0  Capacitance=1e-6  Setx0=off  InitialVoltage=0  Measurements=None
  Subsystem : Subsystem
  Voltage Measurement : spsVoltageMeasurementLib/Voltage Measurement  PhasorSimulation=off  OutputType=Complex  PSBequivalent=0
  car + : PMIOPort  Side=Left
  car - : PMIOPort  Port=2  Side=Left
  tag scope: current_4=global, temperature_4=global, voltage_4=global
  wires:
  Current Measurement/1 -> [current_4], Display1/1
  Voltage Measurement/1 -> [voltage_4], Display/1
  Constant/1 -> [temperature_4]
  connections:
  Series RLC Branch/RConn1 -- Subsystem/LConn2 -- car -/RConn1 -- Voltage Measurement/LConn2
  Series RLC Branch/LConn1 -- Current Measurement/RConn1 -- Voltage Measurement/LConn1
  Current Measurement/LConn1 -- Subsystem/LConn1 -- car +/RConn1

== system SRM_IOT/Subsystem5 ==
  Constant : Constant  Value=300
  Display : Display
  Subsystem : Subsystem
  Voltage Measurement : spsVoltageMeasurementLib/Voltage Measurement  PhasorSimulation=off  OutputType=Complex  PSBequivalent=0
  car + : PMIOPort  Side=Left
  car - : PMIOPort  Port=2  Side=Left
  tag scope: temperature_1=global, voltage_1=global
  wires:
  Voltage Measurement/1 -> [voltage_1], Display/1
  Constant/1 -> [temperature_1]
  connections:
  Subsystem/LConn2 -- Voltage Measurement/LConn2 -- car -/RConn1
  Subsystem/LConn1 -- Voltage Measurement/LConn1 -- car +/RConn1

== system SRM_IOT/Subsystem6 ==
  Constant : Constant  Value=300
  Current Measurement : spsCurrentMeasurementLib/Current Measurement  PhasorSimulation=off  OutputType=Complex  PSBequivalent=0
  Display : Display
  Display1 : Display
  Series RLC Branch : spsSeriesRLCBranchLib/Series RLC Branch  LConnTagsString=__new0  RConnTagsString=__new0  BranchType=R  Resistance=5  Inductance=1e-3  SetiL0=off  InitialCurrent=0  Capacitance=1e-6  Setx0=off  InitialVoltage=0  Measurements=None
  Subsystem : Subsystem
  Voltage Measurement : spsVoltageMeasurementLib/Voltage Measurement  PhasorSimulation=off  OutputType=Complex  PSBequivalent=0
  car + : PMIOPort  Side=Left
  car - : PMIOPort  Port=2  Side=Left
  tag scope: current_2=global, temperature_2=global, voltage_2=global
  wires:
  Current Measurement/1 -> [current_2], Display1/1
  Voltage Measurement/1 -> [voltage_2], Display/1
  Constant/1 -> [temperature_2]
  connections:
  Series RLC Branch/RConn1 -- Subsystem/LConn2 -- car -/RConn1 -- Voltage Measurement/LConn2
  Series RLC Branch/LConn1 -- Current Measurement/RConn1 -- Voltage Measurement/LConn1
  Current Measurement/LConn1 -- Subsystem/LConn1 -- car +/RConn1

== system SRM_IOT/Subsystem7 ==
  Constant : Constant  Value=300
  Current Measurement : spsCurrentMeasurementLib/Current Measurement  PhasorSimulation=off  OutputType=Complex  PSBequivalent=0
  Display : Display
  Display1 : Display
  Series RLC Branch : spsSeriesRLCBranchLib/Series RLC Branch  LConnTagsString=__new0  RConnTagsString=__new0  BranchType=R  Resistance=5  Inductance=1e-3  SetiL0=off  InitialCurrent=0  Capacitance=1e-6  Setx0=off  InitialVoltage=0  Measurements=None
  Subsystem : Subsystem
  Voltage Measurement : spsVoltageMeasurementLib/Voltage Measurement  PhasorSimulation=off  OutputType=Complex  PSBequivalent=0
  car + : PMIOPort  Side=Left
  car - : PMIOPort  Port=2  Side=Left
  tag scope: current_3=global, temperature_3=global, voltage_3=global
  wires:
  Current Measurement/1 -> [current_3], Display1/1
  Voltage Measurement/1 -> [voltage_3], Display/1
  Constant/1 -> [temperature_3]
  connections:
  Series RLC Branch/RConn1 -- Subsystem/LConn2 -- car -/RConn1 -- Voltage Measurement/LConn2
  Series RLC Branch/LConn1 -- Current Measurement/RConn1 -- Voltage Measurement/LConn1
  Current Measurement/LConn1 -- Subsystem/LConn1 -- car +/RConn1

== system SRM_IOT/Subsystem8 ==
  BS + : PMIOPort  Side=Right
  BS - : PMIOPort  Port=2  Side=Right
  FC + : PMIOPort  Port=3  Side=Right
  FC - : PMIOPort  Port=4  Side=Right
  Charger + : PMIOPort  Port=5  Side=Left
  Charger - : PMIOPort  Port=6  Side=Left
  connections:
  FC -/RConn1 -- BS -/RConn1 -- Charger -/RConn1
  FC +/RConn1 -- BS +/RConn1 -- Charger +/RConn1

== system SRM_IOT/Vechicle BMS Monitoring ==
  BMS Discharge : Subsystem
  Saturation : Saturate  UpperLimit=+inf  LowerLimit=0
  wires:
  Saturation/1 -> BMS Discharge/3(Current)
  [current_4] -> Saturation/1
  [terminalvoltage_4] -> BMS Discharge/1(Terminal voltage)
  [temperature_4] -> BMS Discharge/2(Temperature)

== system SRM_IOT/Vechicle BMS Monitoring1 ==
  BMS Discharge : Subsystem
  Saturation : Saturate  UpperLimit=+inf  LowerLimit=0
  wires:
  Saturation/1 -> BMS Discharge/3(Current)
  [current_1] -> Saturation/1
  [terminalvoltage_1] -> BMS Discharge/1(Terminal voltage)
  [temperature_1] -> BMS Discharge/2(Temperature)

== system SRM_IOT/Vechicle BMS Monitoring2 ==
  BMS Discharge : Subsystem
  Saturation : Saturate  UpperLimit=+inf  LowerLimit=0
  wires:
  Saturation/1 -> BMS Discharge/3(Current)
  [current_1] -> Saturation/1
  [terminalvoltage_1] -> BMS Discharge/1(Terminal voltage)
  [temperature_1] -> BMS Discharge/2(Temperature)

== system SRM_IOT/Vechicle BMS Monitoring3 ==
  BMS Discharge : Subsystem
  Saturation : Saturate  UpperLimit=+inf  LowerLimit=0
  wires:
  Saturation/1 -> BMS Discharge/3(Current)
  [current_3] -> Saturation/1
  [terminalvoltage_3] -> BMS Discharge/1(Terminal voltage)
  [temperature_3] -> BMS Discharge/2(Temperature)

== system SRM_IOT/DC//DC converter/DC - DC Converter ==
  C : spsSeriesRLCBranchLib/Series RLC Branch  LConnTagsString=__new0  RConnTagsString=__new0  BranchType=C  Resistance=0.01  Inductance=1e-3  SetiL0=off  InitialCurrent=0  Capacitance=1000e-6  Setx0=on  InitialVoltage=200  Measurements=None
  Diode : spsDiodeLib/Diode  Ron=0.001  Lon=0  Vf=1.1  IC=0  UseSnubber=off  Rs=500  Cs=250e-9  Measurements=off
  Diode2 : spsDiodeLib/Diode  Ron=0.001  Lon=0  Vf=0.7  IC=0  UseSnubber=off  Rs=500  Cs=250e-9  Measurements=off
  IGBT : spsIGBTLib/IGBT  Ron=0.001  Lon=0  Vf=1.1  Tf=1e-6  Tt=2e-6  IC=0  Rs=1e5  Cs=inf  Measurements=off
  RL : spsSeriesRLCBranchLib/Series RLC Branch  LConnTagsString=__new0  RConnTagsString=__new0  BranchType=RL  Resistance=0.05  Inductance=470e-6  SetiL0=off  InitialCurrent=0  Capacitance=1e-6  Setx0=off  InitialVoltage=0  Measurements=None
  DC + : PMIOPort  Side=Right
  solar panel + : PMIOPort  Port=2  Side=Left
  solar panel - : PMIOPort  Port=3  Side=Left
  DC - : PMIOPort  Port=4  Side=Right
  wires:
  [Pulse_PV] -> IGBT/1
  connections:
  Diode/RConn1 -- DC +/RConn1
  Diode2/RConn1 -- C/LConn1 -- RL/LConn1
  Diode/LConn1 -- RL/RConn1 -- IGBT/LConn1
  solar panel +/RConn1 -- Diode2/LConn1
  C/RConn1 -- solar panel -/RConn1 -- DC -/RConn1 -- IGBT/RConn1

== system SRM_IOT/DC//DC converter/DC bus ==
  1 ohm 2000uH : spsSeriesRLCBranchLib/Series RLC Branch  LConnTagsString=__new0  RConnTagsString=__new0  BranchType=RC  Resistance=1  Inductance=0  SetiL0=off  InitialCurrent=0  Capacitance=2000e-6  Setx0=on  InitialVoltage=370  Measurements=None
  RL + : spsSeriesRLCBranchLib/Series RLC Branch  LConnTagsString=__new0  RConnTagsString=__new0  BranchType=RL  Resistance=0.05  Inductance=470e-6  SetiL0=off  InitialCurrent=0  Capacitance=1e-6  Setx0=off  InitialVoltage=0  Measurements=None
  RL - : spsSeriesRLCBranchLib/Series RLC Branch  LConnTagsString=__new0  RConnTagsString=__new0  BranchType=RL  Resistance=0.05  Inductance=470e-6  SetiL0=off  InitialCurrent=0  Capacitance=1e-6  Setx0=off  InitialVoltage=0  Measurements=None
  Transfer Fcn : TransferFcn  Denominator=[1e-4 1]
  V : spsVoltageMeasurementLib/Voltage Measurement  PhasorSimulation=off  OutputType=Complex  PSBequivalent=0
  left + : PMIOPort  Side=Left
  left - : PMIOPort  Port=2  Side=Left
  right + : PMIOPort  Port=3  Side=Right
  right - : PMIOPort  Port=4  Side=Right
  tag scope: Vdc=global
  wires:
  V/1 -> Transfer Fcn/1
  Transfer Fcn/1 -> [Vdc]
  connections:
  RL +/RConn1 -- 1 ohm 2000uH/LConn1 -- right +/RConn1 -- V/LConn1
  RL -/RConn1 -- 1 ohm 2000uH/RConn1 -- right -/RConn1 -- V/LConn2
  left +/RConn1 -- RL +/LConn1
  left -/RConn1 -- RL -/LConn1

== system SRM_IOT/Fast charging controller/Fast charging Switching controller ==
  g1 : Subsystem
  g2 : Subsystem
  g3 : Subsystem
  g4 : Subsystem

== system SRM_IOT/Grid/Wall charger Connection Box ==
  Control : Inport
  Battery Switching Control : Subsystem
      settings: PortSchema="{\"entries\":[{\"content\":{\"sides\":[{\"content\":{\"connectorIds\":[\"LConn1\",\"LConn2\",\"LConn3\",\"LConn4\"]},\"type\":\"ConnectorPlacement.EquallySpacedRectSide\",\"uuid\":\"597ce45f-d2da-489f-9702-c83ae9b1152a\"},{\"content\":{\"connectorIds\":[\"In1\",\"RConn1\",\"RConn2\"],\"side\":\"RIGHT\"},\"type\":\"ConnectorPlacement.EquallySpacedRectSide\",\"uuid\":\"90ab1945-2787-45d6-b647-1c8eb49fe34d\"},{\"content\":{\"connectorIds\":[],\"side\":\"TOP\"},\"type\":\"ConnectorPlacement.EquallySpacedRectSide\",\"uuid\":\"5514c8fd-a1bb-4ed7-b1c0-08bce6a0e9e5\"}]},\"type\":\"ConnectorPlacement.EquallySpacedConnector\",\"uuid\":\"b6d566cb-31ba-40ab-ae9a-003997b713cb\"}],\"packageUris\":[\"http://schema.mathworks.com/mf0/Connector/R2020b\"],\"version\":\"1.0\"}"
  Buck-Boost Converter : Subsystem
  Connection Control : Subsystem
      settings: PortSchema="{\"entries\":[{\"content\":{\"sides\":[{\"content\":{\"connectorIds\":[\"LConn1\",\"LConn2\",\"LConn3\"]},\"type\":\"ConnectorPlacement.EquallySpacedRectSide\",\"uuid\":\"27ebf5cb-61b2-431e-8de2-c9344a0dfca5\"},{\"content\":{\"connectorIds\":[\"In1\",\"RConn1\",\"RConn2\",\"RConn3\",\"RConn4\",\"RConn5\",\"RConn6\"],\"side\":\"RIGHT\"},\"type\":\"ConnectorPlacement.EquallySpacedRectSide\",\"uuid\":\"2438100a-e43b-42f7-afa1-1af449516139\"},{\"content\":{\"connectorIds\":[],\"side\":\"TOP\"},\"type\":\"ConnectorPlacement.EquallySpacedRectSide\",\"uuid\":\"dcfa608d-f6dc-42e3-abf8-45a08af22825\"}]},\"type\":\"ConnectorPlacement.EquallySpacedConnector\",\"uuid\":\"5f0f36e8-f735-4489-a6f2-39fec655b509\"}],\"packageUris\":[\"http://schema.mathworks.com/mf0/Connector/R2020b\"],\"version\":\"1.0\"}"
  DC-AC / AC-DC Converter : Subsystem
  DC-DC converter with battery controller : Subsystem
  Grid_R : PMIOPort  Side=Left
  Grid_Y : PMIOPort  Port=2  Side=Left
  Grid_B : PMIOPort  Port=3  Side=Left
  Vehicle+ : PMIOPort  Port=4  Side=Right
  Vehicle- : PMIOPort  Port=5  Side=Right
  wires:
  Control/1 -> Connection Control/1(Control), Battery Switching Control/1(Control)
  connections:
  DC-AC / AC-DC Converter/LConn5 -- Connection Control/RConn5
  DC-AC / AC-DC Converter/LConn2 -- Connection Control/RConn2
  DC-DC converter with battery controller/RConn3 -- Battery Switching Control/LConn3
  Buck-Boost Converter/RConn2 -- DC-DC converter with battery controller/LConn2
  Grid_B/RConn1 -- Connection Control/LConn3
  DC-AC / AC-DC Converter/RConn3 -- Buck-Boost Converter/LConn3
  Grid_R/RConn1 -- Connection Control/LConn1
  DC-AC / AC-DC Converter/LConn1 -- Connection Control/RConn1
  Vehicle-/RConn1 -- Battery Switching Control/RConn2
  Vehicle+/RConn1 -- Battery Switching Control/RConn1
  Buck-Boost Converter/RConn4 -- DC-DC converter with battery controller/LConn4
  Grid_Y/RConn1 -- Connection Control/LConn2
  DC-AC / AC-DC Converter/LConn4 -- Connection Control/RConn4
  DC-DC converter with battery controller/RConn2 -- Battery Switching Control/LConn2
  DC-DC converter with battery controller/RConn1 -- Battery Switching Control/LConn1
  DC-DC converter with battery controller/RConn4 -- Battery Switching Control/LConn4
  Buck-Boost Converter/RConn1 -- DC-DC converter with battery controller/LConn1
  Buck-Boost Converter/LConn2 -- DC-AC / AC-DC Converter/RConn2
  DC-AC / AC-DC Converter/LConn3 -- Connection Control/RConn3
  DC-AC / AC-DC Converter/RConn1 -- Buck-Boost Converter/LConn1
  DC-AC / AC-DC Converter/RConn4 -- Buck-Boost Converter/LConn4
  Buck-Boost Converter/RConn3 -- DC-DC converter with battery controller/LConn3
  Connection Control/RConn6 -- DC-AC / AC-DC Converter/LConn6

== system SRM_IOT/MPPT and PV Controller/Inverter controller ==
  Constant1 : Constant  Value=370
  Inverter Controller : Subsystem
  Transfer Fcn1 : TransferFcn  Denominator=[1e-5 1]
  Transfer Fcn8 : TransferFcn  Denominator=[1e-5 1]
  tag scope: Pulse_UI=global
  wires:
  Inverter Controller/1(Pulse) -> [Pulse_UI]
  Constant1/1 -> Inverter Controller/2(370)
  [I_Sys_Secondary] -> Transfer Fcn1/1
  Transfer Fcn1/1 -> Inverter Controller/4(I_Sys_Secondary)
  [Grid_Connection_ON] -> Inverter Controller/Enable
  [V_Sys_Secondary] -> Inverter Controller/3(V_Sys_Secondary)
  [Vdc] -> Transfer Fcn8/1
  Transfer Fcn8/1 -> Inverter Controller/1(V_Dc)

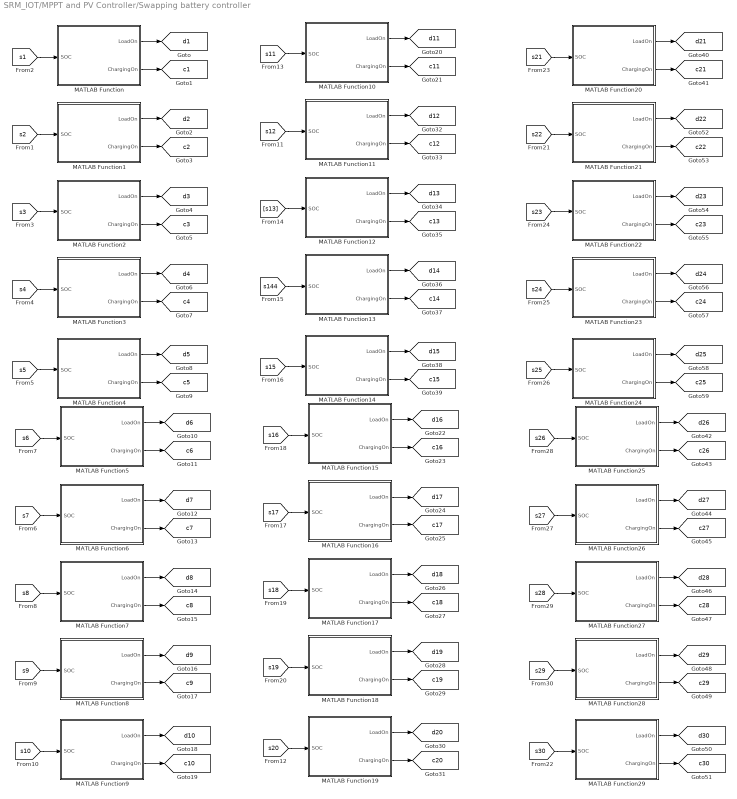
== system SRM_IOT/MPPT and PV Controller/Swapping battery controller ==
  MATLAB Function : MATLAB Function  TreatAsAtomicUnit=on
  MATLAB Function1 : MATLAB Function  TreatAsAtomicUnit=on
  MATLAB Function10 : MATLAB Function  TreatAsAtomicUnit=on
  MATLAB Function11 : MATLAB Function  TreatAsAtomicUnit=on
  MATLAB Function12 : MATLAB Function  TreatAsAtomicUnit=on
  MATLAB Function13 : MATLAB Function  TreatAsAtomicUnit=on
  MATLAB Function14 : MATLAB Function  TreatAsAtomicUnit=on
  MATLAB Function15 : MATLAB Function  TreatAsAtomicUnit=on
  MATLAB Function16 : MATLAB Function  TreatAsAtomicUnit=on
  MATLAB Function17 : MATLAB Function  TreatAsAtomicUnit=on
  MATLAB Function18 : MATLAB Function  TreatAsAtomicUnit=on
  MATLAB Function19 : MATLAB Function  TreatAsAtomicUnit=on
  MATLAB Function2 : MATLAB Function  TreatAsAtomicUnit=on
  MATLAB Function20 : MATLAB Function  TreatAsAtomicUnit=on
  MATLAB Function21 : MATLAB Function  TreatAsAtomicUnit=on
  MATLAB Function22 : MATLAB Function  TreatAsAtomicUnit=on
  MATLAB Function23 : MATLAB Function  TreatAsAtomicUnit=on
  MATLAB Function24 : MATLAB Function  TreatAsAtomicUnit=on
  MATLAB Function25 : MATLAB Function  TreatAsAtomicUnit=on
  MATLAB Function26 : MATLAB Function  TreatAsAtomicUnit=on
  MATLAB Function27 : MATLAB Function  TreatAsAtomicUnit=on
  MATLAB Function28 : MATLAB Function  TreatAsAtomicUnit=on
  MATLAB Function29 : MATLAB Function  TreatAsAtomicUnit=on
  MATLAB Function3 : MATLAB Function  TreatAsAtomicUnit=on
  MATLAB Function4 : MATLAB Function  TreatAsAtomicUnit=on
  MATLAB Function5 : MATLAB Function  TreatAsAtomicUnit=on
  MATLAB Function6 : MATLAB Function  TreatAsAtomicUnit=on
  MATLAB Function7 : MATLAB Function  TreatAsAtomicUnit=on
  MATLAB Function8 : MATLAB Function  TreatAsAtomicUnit=on
  MATLAB Function9 : MATLAB Function  TreatAsAtomicUnit=on
  tag scope: c10=global, c11=global, c12=global, c13=global, c14=global, c15=global, c16=global, c17=global, c18=global, c19=global, c1=global, c20=global, c21=global, c22=global, c23=global, c24=global, c25=global, c26=global, c27=global, c28=global, c29=global, c2=global, c30=global, c3=global, c4=global, c5=global, c6=global, c7=global, c8=global, c9=global, d10=global, d11=global, d12=global, d13=global, d14=global, d15=global, d16=global, d17=global, d18=global, d19=global, d1=global, d20=global, d21=global, d22=global, d23=global, d24=global, d25=global, d26=global, d27=global, d28=global, d29=global, d2=global, d30=global, d3=global, d4=global, d5=global, d6=global, d7=global, d8=global, d9=global
  wires:
  MATLAB Function10/1(LoadOn) -> [d11]
  MATLAB Function1/2(ChargingOn) -> [c2]
  [s20] -> MATLAB Function19/1(SOC)
  [s22] -> MATLAB Function21/1(SOC)
  MATLAB Function5/1(LoadOn) -> [d6]
  [s16] -> MATLAB Function15/1(SOC)
  [s5] -> MATLAB Function4/1(SOC)
  MATLAB Function/2(ChargingOn) -> [c1]
  MATLAB Function2/2(ChargingOn) -> [c3]
  MATLAB Function26/1(LoadOn) -> [d27]
  [s21] -> MATLAB Function20/1(SOC)
  MATLAB Function18/1(LoadOn) -> [d19]
  MATLAB Function7/2(ChargingOn) -> [c8]
  MATLAB Function12/2(ChargingOn) -> [c13]
  MATLAB Function28/1(LoadOn) -> [d29]
  MATLAB Function4/2(ChargingOn) -> [c5]
  MATLAB Function25/2(ChargingOn) -> [c26]
  [s1] -> MATLAB Function/1(SOC)
  MATLAB Function11/2(ChargingOn) -> [c12]
  MATLAB Function/1(LoadOn) -> [d1]
  MATLAB Function16/1(LoadOn) -> [d17]
  MATLAB Function10/2(ChargingOn) -> [c11]
  [s15] -> MATLAB Function14/1(SOC)
  [s12] -> MATLAB Function11/1(SOC)
  [s3] -> MATLAB Function2/1(SOC)
  MATLAB Function2/1(LoadOn) -> [d3]
  MATLAB Function17/1(LoadOn) -> [d18]
  MATLAB Function13/2(ChargingOn) -> [c14]
  MATLAB Function4/1(LoadOn) -> [d5]
  MATLAB Function14/2(ChargingOn) -> [c15]
  MATLAB Function3/1(LoadOn) -> [d4]
  MATLAB Function6/2(ChargingOn) -> [c7]
  [s7] -> MATLAB Function6/1(SOC)
  MATLAB Function15/1(LoadOn) -> [d16]
  MATLAB Function26/2(ChargingOn) -> [c27]
  [s8] -> MATLAB Function7/1(SOC)
  MATLAB Function6/1(LoadOn) -> [d7]
  MATLAB Function13/1(LoadOn) -> [d14]
  MATLAB Function16/2(ChargingOn) -> [c17]
  MATLAB Function18/2(ChargingOn) -> [c19]
  MATLAB Function5/2(ChargingOn) -> [c6]
  [s6] -> MATLAB Function5/1(SOC)
  [s18] -> MATLAB Function17/1(SOC)
  [s13] -> MATLAB Function12/1(SOC)
  MATLAB Function19/2(ChargingOn) -> [c20]
  MATLAB Function22/1(LoadOn) -> [d23]
  [s27] -> MATLAB Function26/1(SOC)
  MATLAB Function19/1(LoadOn) -> [d20]
  [s26] -> MATLAB Function25/1(SOC)
  [s29] -> MATLAB Function28/1(SOC)
  MATLAB Function8/2(ChargingOn) -> [c9]
  [s17] -> MATLAB Function16/1(SOC)
  MATLAB Function17/2(ChargingOn) -> [c18]
  [s19] -> MATLAB Function18/1(SOC)
  MATLAB Function3/2(ChargingOn) -> [c4]
  MATLAB Function11/1(LoadOn) -> [d12]
  [s11] -> MATLAB Function10/1(SOC)
  MATLAB Function8/1(LoadOn) -> [d9]
  [s2] -> MATLAB Function1/1(SOC)
  MATLAB Function12/1(LoadOn) -> [d13]
  [s10] -> MATLAB Function9/1(SOC)
  MATLAB Function14/1(LoadOn) -> [d15]
  [s144] -> MATLAB Function13/1(SOC)
  MATLAB Function1/1(LoadOn) -> [d2]
  [s4] -> MATLAB Function3/1(SOC)
  MATLAB Function15/2(ChargingOn) -> [c16]
  MATLAB Function7/1(LoadOn) -> [d8]
  [s9] -> MATLAB Function8/1(SOC)
  MATLAB Function9/1(LoadOn) -> [d10]
  MATLAB Function9/2(ChargingOn) -> [c10]
  MATLAB Function29/2(ChargingOn) -> [c30]
  MATLAB Function29/1(LoadOn) -> [d30]
  MATLAB Function27/2(ChargingOn) -> [c28]
  MATLAB Function25/1(LoadOn) -> [d26]
  [s28] -> MATLAB Function27/1(SOC)
  [s30] -> MATLAB Function29/1(SOC)
  MATLAB Function28/2(ChargingOn) -> [c29]
  MATLAB Function23/1(LoadOn) -> [d24]
  [s24] -> MATLAB Function23/1(SOC)
  MATLAB Function23/2(ChargingOn) -> [c24]
  MATLAB Function21/1(LoadOn) -> [d22]
  MATLAB Function27/1(LoadOn) -> [d28]
  MATLAB Function24/1(LoadOn) -> [d25]
  MATLAB Function22/2(ChargingOn) -> [c23]
  [s23] -> MATLAB Function22/1(SOC)
  MATLAB Function24/2(ChargingOn) -> [c25]
  [s25] -> MATLAB Function24/1(SOC)
  MATLAB Function20/2(ChargingOn) -> [c21]
  MATLAB Function21/2(ChargingOn) -> [c22]
  MATLAB Function20/1(LoadOn) -> [d21]

== system SRM_IOT/Solar/Irradiance  ==
  Demux : Demux  Tag=STV Demux  Outputs=2
      settings: DisplayOption=none
  FromWs : FromWorkspace  Tag=STV FromWs  VariableName=tuvar
      SigBuilderData=|
      | common.afterFinalStr = 'Extrapolate'
      | common.sampleTime = '0'
      | dataSet(1).timeRange = [0 2]
      | dataSet(1).name = 'Constant Irradiance'
      | dataSet(2).timeRange = [0 2]
      | dataSet(2).name = 'Step Irradiance'
      | dataSet(3).timeRange = [0 1]
      | dataSet(3).name = 'Ramp-up/down Irradiance'
      | sbobj.Groups(1).Name = 'Constant Irradiance'
      | sbobj.Groups(1).Signals(1).Name = 'Ir'
      | sbobj.Groups(1).Signals(1).XData = [0 2]
      | sbobj.Groups(1).Signals(1).YData = [1000 1000]
      | sbobj.Groups(1).Signals(2).Name = 'Temp'
      | sbobj.Groups(1).Signals(2).XData = [0 1 1 2]
      | sbobj.Groups(1).Signals(2).YData = [0 0 1 1]
      | sbobj.Groups(1).TimeRange = [0 2]
      | sbobj.Groups(2).Name = 'Step Irradiance'
      | sbobj.Groups(2).Signals(1).Name = 'Ir'
      | sbobj.Groups(2).Signals(1).XData = [0 0.252 0.252 2]
      | sbobj.Groups(2).Signals(1).YData = [600 600 1000 1000]
      | sbobj.Groups(2).Signals(2).Name = 'Temp'
      | sbobj.Groups(2).Signals(2).XData = [0 1 1 2]
      | sbobj.Groups(2).Signals(2).YData = [0 0 1 1]
      | sbobj.Groups(2).TimeRange = [0 2]
      | sbobj.Groups(3).Name = 'Ramp-up/down Irradiance'
      | sbobj.Groups(3).Signals(1).Name = 'Ir'
      | sbobj.Groups(3).Signals(1).XData = [0 0.3 0.3 0.4 0.4 0.5 0.5 1]
      | sbobj.Groups(3).Signals(1).YData = [1000 1000 800 795 600 600 400 395]
      | sbobj.Groups(3).Signals(2).Name = 'Temp'
      | sbobj.Groups(3).Signals(2).XData = [0 1]
      | sbobj.Groups(3).Signals(2).YData = [25 25]
      | sbobj.Groups(3).TimeRange = [0 1]
  Ir : Outport  Tag=STV Outport
  Temp : Outport  Tag=STV Outport  Port=2
  wires:
  Demux/1 -> Ir/1
  FromWs/1 -> Demux/1
  Demux/2 -> Temp/1

== system SRM_IOT/Solar/MPPT ==
  "V _ PV " : Inport
  I_PV : Inport  Port=2
  clock : Inport  Port=3
  Embedded MATLAB Function1 : MATLAB Function  TreatAsAtomicUnit=on
  Duty : Outport  VectorParamsAs1DForOutWhenUnconnected=off
  wires:
  Embedded MATLAB Function1/1(D) -> Duty/1
  clock/1 -> Embedded MATLAB Function1/3(T)
  "V _ PV "/1 -> Embedded MATLAB Function1/1(V)
  I_PV/1 -> Embedded MATLAB Function1/2(I)
